simulink model "UnlinearSimulationArmContollerOnly"  (R2017a)
settings: Solver=VariableStepAuto  StartTime=0.0  StopTime=10.0  RelTol=1e-3
libraries: simulink x1
settings Model: Creator=khrom  LastModifiedBy=khrom

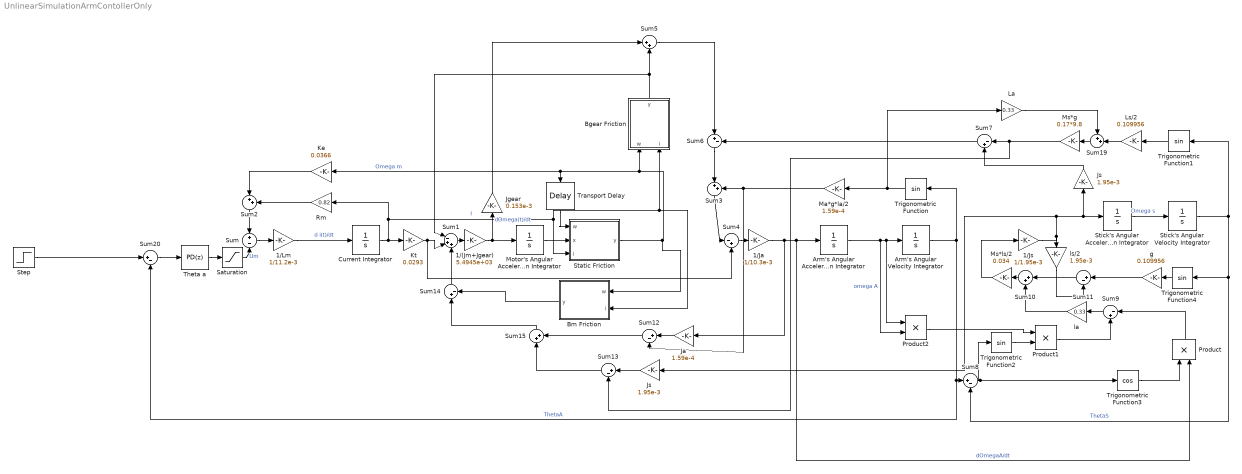
== system UnlinearSimulationArmContollerOnly ==
  1/(Jm+Jgear) : Gain  Gain=5.4945e+03
  1/Ja : Gain  Gain=1/10.3e-3
  1/Js : Gain  Gain=1/1.95e-3
  1/Lm : Gain  Gain=1/11.2e-3
  Arm's Angular Acceleration Integrator : TransferFcn  Denominator=[1 0]
  Arm's Angular Velocity Integrator : TransferFcn  Denominator=[1 0]
  Bgear Friction : MATLAB Function  TreatAsAtomicUnit=on
  Bm Friction : MATLAB Function  TreatAsAtomicUnit=on
  Current Integrator : TransferFcn  Denominator=[1 0]
  Ja : Gain  Gain=1.59e-4
  Jgear : Gain  Gain=0.153e-3
  Js : Gain  Gain=1.95e-3
  "Js " : Gain  Gain=1.95e-3
  Ke : Gain  Gain=0.0366
  Kt : Gain  Gain=0.0293
  La : Gain  Gain=0.33
  Ls/2 : Gain  Gain=0.109956
  Ma*g*la/2 : Gain  Gain=1.59e-4
  Motor's Angular Acceleration Integrator : TransferFcn  Denominator=[1 0]
  Ms*g : Gain  Gain=0.17*9.8
  Ms*ls/2 : Gain  Gain=0.034
  Product : Product
  Product1 : Product
  Product2 : Product
  Rm : Gain  Gain=0.82
  Saturation : Saturate  UpperLimit=14  LowerLimit=-14
  Static Friction : MATLAB Function  TreatAsAtomicUnit=on
  Step : Step  Time=0  SampleTime=10*pi/180
  Stick's Angular Acceleration Integrator : TransferFcn  Denominator=[1 0]
  Stick's Angular Velocity Integrator : TransferFcn  Denominator=[1 0]
  Sum : Sum  Inputs=+-
  Sum1 : Sum  Inputs=|-++
  Sum{2..3,5,10,15} (5 alike) : Sum  Inputs=|++
  Sum{6,8,11..14,20} (7 alike) : Sum  Inputs=|+-
  Sum19 : Sum  Inputs=++|
  Sum4 : Sum  Inputs=|-+
  Sum7 : Sum  Inputs=|-+
  Sum9 : Sum  Inputs=|-+
  Theta a : simulink/Continuous/PID Controller  Controller=PD  TimeDomain=Discrete-time  SampleTime=-1  IntegratorMethod=Forward Euler  FilterMethod=Forward Euler  Form=Parallel  UseFilter=on  ControllerParametersSource=internal  P=609  I=0  D=9  N=100  InitialConditionSource=internal  InitialConditionForIntegrator=0  InitialConditionForFilter=0  ExternalReset=none  LimitOutput=off  UpperSaturationLimit=inf  LowerSaturationLimit=-inf  LinearizeAsGain=on  AntiWindupMode=none  Kb=1  TrackingMode=off  Kt=1  PParamMin=[]  PParamMax=[]  IParamMin=[]  IParamMax=[]  DParamMin=[]  DParamMax=[]  NParamMin=[]  NParamMax=[]  KbParamMin=[]  KbParamMax=[]  KtParamMin=[]  KtParamMax=[]  POutMin=[]  POutMax=[]  IOutMin=[]  IOutMax=[]  DOutMin=[]  DOutMax=[]  NOutMin=[]  NOutMax=[]  KbOutMin=[]  KbOutMax=[]  KtOutMin=[]  KtOutMax=[]  IntegratorOutMin=[]  IntegratorOutMax=[]  FilterOutMin=[]  FilterOutMax=[]  SumOutMin=[]  SumOutMax=[]  SumI1OutMin=[]  SumI1OutMax=[]  SumI2OutMin=[]  SumI2OutMax=[]  SumI3OutMin=[]  SumI3OutMax=[]  SumDOutMin=[]  SumDOutMax=[]  SaturationOutMin=[]  SaturationOutMax=[]  IntegratorContinuousStateAttributes=''  IntegratorStateMustResolveToSignalObject=off  IntegratorRTWStateStorageClass=Auto  FilterContinuousStateAttributes=''  FilterStateMustResolveToSignalObject=off  FilterRTWStateStorageClass=Auto  DifferentiatorICPrevScaledInput=0  DifferentiatorOutMin=[]  DifferentiatorOutMax=[]  InitialConditionSetting=State (most efficient)
  Transport Delay : TransportDelay  DelayTime=0.000000000000000000000000001
  Trigonometric Function{,1..2,4} (4 alike) : Trigonometry
  Trigonometric Function3 : Trigonometry  Operator=cos
  g : Gain  Gain=0.109956
  la : Gain  Gain=0.33
  ls/2 : Gain  Gain=1.95e-3
  wires:
  Arm's Angular Acceleration Integrator/1 -> Product2/2, Arm's Angular Velocity Integrator/1, Product2/1  "omega A"
  Stick's Angular Acceleration Integrator/1 -> Stick's Angular Velocity Integrator/1  "Omega s"
  Current Integrator/1 -> Static Friction/3(i), Bm Friction/2(i), Bgear Friction/2(i), Rm/1, Kt/1  "I"
  Theta a/1 -> Saturation/1
  Sum/1 -> 1/Lm/1
  1/Lm/1 -> Current Integrator/1  "d i(t)/dt"
  Sum2/1 -> Sum/1
  Rm/1 -> Sum2/2
  Ke/1 -> Sum2/1
  1/(Jm+Jgear)/1 -> Motor's Angular Acceleration Integrator/1, Jgear/1  "dOmega(t)/dt"
  Kt/1 -> Sum1/2, Sum4/2
  1/Ja/1 -> Ja/1, Product/2, Arm's Angular Acceleration Integrator/1  "dOmegaA/dt"
  Arm's Angular Velocity Integrator/1 -> Sum20/2, Sum8/1, Trigonometric Function/1  "ThetaA"
  Trigonometric Function/1 -> La/1, Ma*g*la/2/1
  Ma*g*la/2/1 -> Sum12/2, Sum3/2
  Sum3/1 -> Sum4/1
  Sum4/1 -> 1/Ja/1
  Jgear/1 -> Sum5/1
  Sum5/1 -> Sum6/1
  Sum6/1 -> Sum3/1
  1/Js/1 -> ls/2/1, "Js "/1, Js/1, Stick's Angular Acceleration Integrator/1
  Js/1 -> Sum7/2
  Ms*g/1 -> Sum13/2, Sum7/1
  Trigonometric Function1/1 -> Ls/2/1
  Sum7/1 -> Sum6/2
  Stick's Angular Velocity Integrator/1 -> Trigonometric Function4/1, Sum8/2, Trigonometric Function1/1  "ThetaS"
  Trigonometric Function3/1 -> Product/1
  Product/1 -> Sum9/1
  Sum8/1 -> Trigonometric Function2/1, Trigonometric Function3/1
  Trigonometric Function2/1 -> Product1/2
  Product1/1 -> Sum9/2
  Product2/1 -> Product1/1
  Sum9/1 -> la/1
  la/1 -> Sum10/2
  ls/2/1 -> Sum11/2
  Trigonometric Function4/1 -> g/1
  g/1 -> Sum11/1
  Sum11/1 -> Sum10/1
  Sum10/1 -> Ms*ls/2/1
  Ms*ls/2/1 -> 1/Js/1
  Ja/1 -> Sum12/1
  "Js "/1 -> Sum13/1
  Sum14/1 -> Sum1/3
  Bm Friction/1(y) -> Sum14/2
  Sum12/1 -> Sum15/2
  Sum13/1 -> Sum15/1
  Sum15/1 -> Sum14/1
  Sum1/1 -> 1/(Jm+Jgear)/1
  Saturation/1 -> Sum/2  "Um"
  Motor's Angular Acceleration Integrator/1 -> Static Friction/2(x)
  Static Friction/1(y) -> Bm Friction/1(w), Bgear Friction/1(w), Ke/1, Transport Delay/1  "Omega m"
  Bgear Friction/1(y) -> Sum1/1, Sum5/2
  Transport Delay/1 -> Static Friction/1(w)
  Ls/2/1 -> Sum19/2
  Sum19/1 -> Ms*g/1
  Sum20/1 -> Theta a/1
  Step/1 -> Sum20/1
  La/1 -> Sum19/1

== matlab function UnlinearSimulationArmContollerOnly/Static Friction ==
  data: w input; x input; y output; i input
function y = fcn(w,x,i)

Bm=1.59e-4;
imini=0;

if w~=0
    y=x;
elseif i>imini
    y=x;
else
    y=0;
end

== matlab function UnlinearSimulationArmContollerOnly/Bm Friction ==
  data: w input; y output; i input
function y = fcn(w,i)

Bm=1.59e-4;
imini=0;
Kt=0.0293;

if w~=0
    y=Bm*w;
elseif i>imini
    y=Kt*imini;
else
    y=Kt*i;
end

== matlab function UnlinearSimulationArmContollerOnly/Bgear Friction ==
  data: w input; y output; i input
function y = fcn(w,i)

Bgear=1.11e-3;
imini=0;
Kt=0.0293;
N=0.3;

if w~=0
    y=Bgear*w;
elseif i>imini
    y=Kt*imini/N^3;
else
    y=Kt*i/N^3;
end
